simulink model "TZ4_SAU_ElPrivod_Nastr_Reg_Veps01"  (R2022a)
settings: Solver=VariableStepAuto  StartTime=0.0  StopTime=inf  RelTol=1e-3
undefined symbols (not defined in the file): CF, DiscIntNeverNeededParam, DT, Es, FI, Filter, PI_reg, RaLa, ReLe, Rsh0, SAU_ElPrivod, SAU_ElPrivod_Nastr_Reg, TagPr, Tokivx, TP, TS, UravDvij, ZU
libraries: spsSeriesRLCBranchLib x18, spsCurrentMeasurementLib x17, spsControlledVoltageSourceLib x8, spsVoltageMeasurementLib x4, dspsigattribs x2, dspstat3 x2, simulink x2, spsIGBTLib x2, spsIdealSwitchLib x1, dspswit3 x1, spsDiodeLib x1, spsDCVoltageSourceLib x1
(part 1 of 2)
settings Model: Creator=админ  LastModifiedBy=админ

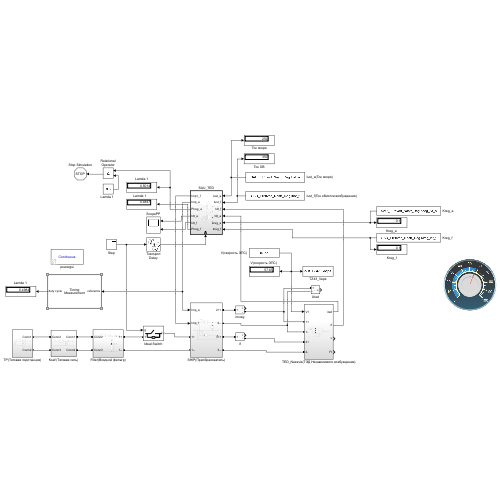
[thumbnail: Simulink's stored preview of the top-level diagram]
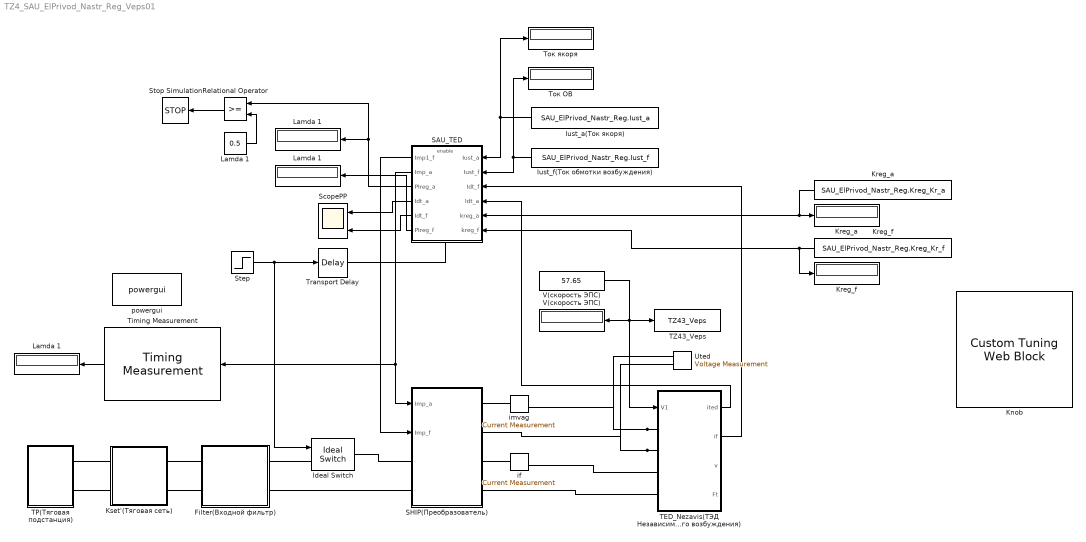
== system TZ4_SAU_ElPrivod_Nastr_Reg_Veps01 ==
  Filter(Входной фильтр) : Subsystem
  Ideal Switch : spsIdealSwitchLib/Ideal Switch  Ron=0.001  Lon=0  IC=0  Rs=1e5  Cs=inf  Measurements=off
  "Iust_a(Ток якоря) " : Constant  Value=SAU_ElPrivod_Nastr_Reg.Iust_a
  Iust_f(Ток обмотки возбуждения) : Constant  Value=SAU_ElPrivod_Nastr_Reg.Iust_f
  Knob : CustomTuningWebBlock  LabelPosition=Hide  ShowInitialText=on  Configuration="{\"components\":[{\"name\":\"CircularScaleComponent\",\"settings\":{\"bounds\":{\"max\":100,\"min\":0,\"tickInterval\":10},\"direction\":\"cw\",\"flipLimits\":0,\"innerRadius\":0.6636618227670849,\"internalTickHeightScaleFactor\":1,\"labelColor\":[255,255,200],\"labelFont\":{\"font\":\"Arial\",\"fontSize\":12},\"labelTransparency\":1,\"minorTickHeightScaleFactor\":0.2,\"needleImage\":{\"size\":[150,150],\"src\":\"data:image\\/svg+xml;base64,PD94bWwgdmVyc2lvbj0iMS4wIiBlbmNvZGluZz0idXRmLTgiPz4NCjwhLS0gR2VuZXJhdG9yOiBBZG9iZSBJbGx1c3RyYXRvciAyNS4yLjMsIFNWRyBFeHBvcnQgUGx1Zy1JbiAuIFNWRyBWZXJzaW9uOiA2LjAwIEJ1aWxkIDApICAtLT4NCjxzdmcgdmVyc2lvbj0iMS4xIiBpZD0iTGF5ZXJfMSIgeG1sbnM9Imh0dHA6Ly93d3cudzMub3JnLzIwMDAvc3ZnIiB4bWxuczp4bGluaz0iaHR0cDovL3d3dy53My5vcmcvMTk5OS94bGluayIgeD0iMHB4IiB5PSIwcHgiDQoJIHZpZXdCb3g9IjAgMCAxNTIgMTUyIiBzdHlsZT0iZW5hYmxl ...(+37472 chars)\"},\"needleOffset\":[0,0],\"needleOrientation\":-45,\"needleRotation\":90,\"needleSize\":{\"height\":0.44,\"width\":0.44},\"outerRadius\":0.5053386200069245,\"position\":[0.004939516129032258,0,1,1],\"referencePoint\":\"auto\",\"scaleAngle\":270,\"scaleAngleOffset\":135,\"scaleColors\":[],\"scaleColorsSize\":0.2,\"scaleDirection\":\"CW\",\"scalePosition\":[0,0,1,1],\"showLabels\":1,\"showMinorTicks\":1,\"showSpanLine\":true,\"showTicks\":1,\"tickColor\":[252,252,197],\"tickTransparency\":1,\"valueBarColor\":[0,114,189],\"valueBarPosition\":[0,0,1,1],\"valueBarSize\":0.2,\"valueBarTransparency\":1}},{\"name\":\"BackgroundImageComponent\",\"settings\":{\"image\":{\"size\":[385,373],\"src\":\"data:image\\/svg+xml;base64,PD94bWwgdmVyc2lvbj0iMS4wIiBlbmNvZGluZz0idXRmLTgiPz4NCjwhLS0gR2VuZXJhdG9yOiBBZG9iZSBJbGx1c3RyYXRvciAyNS4wLjAsIFNWRyBFeHBvcnQgUGx1Zy1JbiAuIFNWRyBWZXJzaW9uOiA2LjAwIEJ1aWxkIDApICAtLT4NCjxzdmcgdmVyc2lvbj0iMS4xIg0KCSBpZD0iTGF5ZXJfMl8xXyIgeG1sbnM6Y2M9Imh0dHA6Ly9jcmVhdGl2ZWNvbW1vbnMub3JnL25zIyIgeG1sbnM6ZGM9Imh0dHA6Ly9wdXJsLm9yZy9kYy9lbGVtZW50cy8xLjEvIiB4bWxuczppbmtzY2FwZT0iaHR0cDovL3d3dy5pbmtzY2FwZS5vcmcv ...(+4184 chars)\",\"srcOrientation\":\"horizontal\"},\"position\":[0,0,1,1],\"scaleMode\":\"0\"}},{\"name\":\"ForegroundImageComponent\",\"settings\":{\"image\":{\"size\":[0,0],\"src\":\"default\",\"srcOrientation\":[]},\"isForeground\":1,\"position\":[0,0,1,1],\"scaleMode\":\"0\"}}],\"settings\":{\"BindingType\":\"param\",\"aspectRatio\":1,\"backgroundColor\":[0,0,0,\"1\"],\"backgroundOffset\":0,\"backgroundOpacity\":1,\"direction\":\"cw\",\"fixedAspectRatio\":\"on\",\"flipLimits\":0,\"foregroundColor\":[252,252,196],\"orientation\":\"horizontal\",\"showBackgroundColor\":false,\"value\":0},\"type\":\"CircularGauge\"}"
  "Kreg_a " : Display
  "Kreg_a  " : Constant  Value=SAU_ElPrivod_Nastr_Reg.Kreg_Kr_a
  Kreg_f : Display
  "Kreg_f " : Constant  Value=SAU_ElPrivod_Nastr_Reg.Kreg_Kr_f
  Kset'(Тяговая сеть) : Subsystem
  Lamda 1 : Display
  "Lamda 1 " : Display
  "Lamda 1  " : Constant  Value=0.5
  "Lamda 1    " : Display
  Relational Operator : RelationalOperator  OutDataTypeStr=boolean  RndMeth=Simplest  InputSameDT=off
  SAU_TED : Subsystem
  SHIP(Преобразователь) : Subsystem
  ScopePP : Scope  NumInputPorts=2
  Step : Step  Time=SAU_ElPrivod.Step_time  SampleTime=0
  Stop Simulation : Stop
  TED_Nezavis(ТЭД Независимого возбуждения) : Subsystem
  TP(Тяговая подстанция) : Subsystem
  TZ43_Veps : ToWorkspace  VariableName=TZ43_Veps  SampleTime=-1
  Timing Measurement : msbUtilities/Timing Measurement  Period=off  Frequency=off  RiseTime=off  FallTime=off  DutyCycle=on  Delay=off  SameRefThreshold=on  GlobalRefThreshold=0  Range=[-1 1]  MeasurementType=80% / 20%  ThresholdMax=0.6  ThresholdMin=-0.6  DcRefThreshold=0  DelayRefThreshold=0  DelayTstThreshold=0
      settings: SourceProductBaseCode=AM
  Transport Delay : TransportDelay
  Uted : spsVoltageMeasurementLib/Voltage Measurement  PhasorSimulation=off  OutputType=Complex  PSBequivalent=0
  V(скорость ЭПС) : Constant  Value=57.65
  "V(скорость ЭПС) " : Display
  if : spsCurrentMeasurementLib/Current Measurement  PhasorSimulation=off  OutputType=Complex  PSBequivalent=0
  imvag : spsCurrentMeasurementLib/Current Measurement  PhasorSimulation=off  OutputType=Complex  PSBequivalent=0
  powergui : spspowerguiLib/powergui  Priority=1  SimulationMode=Continuous  SampleTime=50e-6  frequency=60  Iterations=50  frequencyindice=0  Pbase=100e6  ErrMax=1e-4  UnitsV=kV  UnitsW=MW  buscounter=0  FunctionMessages=off  echomessages=off  EnableUseOfTLC=off  CurrentSourceSwitches=off  DisableSnubberDevices=off  DisableRonSwitches=off  DisableVfSwitches=off  DisplayEquations=off  AutomaticDiscreteSolvers=off  SolverType=Tustin/Backward Euler (TBE)  Interpol=off  ExternalGateDelay=off  methode=off  Ts=100  x0status=blocks  SPID=on  SwTol=0  HookPort=off  NonlinearTolerance=1e-4  nMaxIteration=100  ContinueOnMaxIteration=off  RestoreLinks=warning  ResistiveCurrentMeasurement=off  Frange=[0:2:500]  Ylog=off  Xlog=on  ShowGrid=off  save=off  variable=ZData  structure=0  ZoomFFT=off  StartTime=0.0  cycles=1  DisplayStyle=1  fundamental=60  FreqAxis=off  MaxFrequency=1000  frequencyindicesteady=1  RmsSteady=1  display=off
  Ток ОВ : Display
  Ток якоря : Display
  wires:
  TED_Nezavis(ТЭД Независимого возбуждения)/1(ited) -> SAU_TED/4(Idt_a)
  TED_Nezavis(ТЭД Независимого возбуждения)/2(if) -> SAU_TED/3(Idt_f)
  SAU_TED/1(Imp1_f) -> SHIP(Преобразователь)/2(Imp_f)
  "Iust_a(Ток якоря) "/1 -> SAU_TED/1(Iust_a), Ток якоря/1
  Iust_f(Ток обмотки возбуждения)/1 -> SAU_TED/2(Iust_f), Ток ОВ/1
  Transport Delay/1 -> SAU_TED/Enable
  Step/1 -> Ideal Switch/1, Transport Delay/1
  V(скорость ЭПС)/1 -> TZ43_Veps/1, TED_Nezavis(ТЭД Независимого возбуждения)/1(V1), "V(скорость ЭПС) "/1
  "Kreg_a  "/1 -> SAU_TED/5(kreg_a), "Kreg_a "/1
  SAU_TED/3(PIreg_a) -> Relational Operator/1, Lamda 1/1
  SAU_TED/4("Idt_a ") -> ScopePP/1
  SAU_TED/5("Idt_f ") -> ScopePP/2
  Timing Measurement/1 -> "Lamda 1 "/1
  SAU_TED/2(Imp_a) -> Timing Measurement/1, SHIP(Преобразователь)/1(Imp_a)
  "Lamda 1  "/1 -> Relational Operator/2
  Relational Operator/1 -> Stop Simulation/1
  "Kreg_f "/1 -> Kreg_f/1, SAU_TED/6(kreg_f)
  SAU_TED/6(PIreg_f) -> "Lamda 1    "/1
  connections:
  TED_Nezavis(ТЭД Независимого возбуждения)/LConn2 -- SHIP(Преобразователь)/RConn2 -- Uted/LConn2
  TED_Nezavis(ТЭД Независимого возбуждения)/LConn1 -- imvag/RConn1 -- Uted/LConn1
  if/LConn1 -- SHIP(Преобразователь)/RConn3
  Kset'(Тяговая сеть)/LConn2 -- TP(Тяговая подстанция)/RConn2
  Kset'(Тяговая сеть)/RConn1 -- Filter(Входной фильтр)/LConn1
  imvag/LConn1 -- SHIP(Преобразователь)/RConn1
  if/RConn1 -- TED_Nezavis(ТЭД Независимого возбуждения)/LConn3
  Kset'(Тяговая сеть)/RConn2 -- Filter(Входной фильтр)/LConn2
  TP(Тяговая подстанция)/RConn1 -- Kset'(Тяговая сеть)/LConn1
  SHIP(Преобразователь)/RConn4 -- TED_Nezavis(ТЭД Независимого возбуждения)/LConn4
  SHIP(Преобразователь)/LConn2 -- Filter(Входной фильтр)/RConn2
  Ideal Switch/RConn1 -- SHIP(Преобразователь)/LConn1
  Ideal Switch/LConn1 -- Filter(Входной фильтр)/RConn1
